simulink library "INP_DRVR"  (R2024b)
settings: Solver=VariableStepAuto  StartTime=0.0  StopTime=10.0  RelTol=1e-3
undefined symbols (not defined in the file or in its folder): p_RatSt_na
libraries: INP_DRVR_ManOver x1, INP_DRVR_Prep x1
settings Model: Creator=blatak  LastModifiedBy=jmbsp
settings ModelReferenceCC: EnableRefExpFcnMdlSchedulingChecks=on
settings RTWCC: GPUComputeCapability=3.5

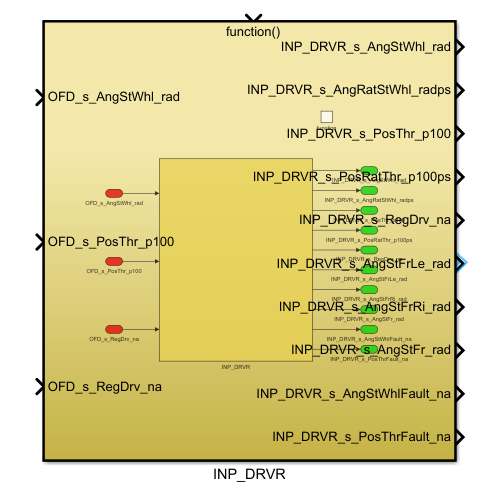
[thumbnail: Simulink's stored preview of the top-level diagram]
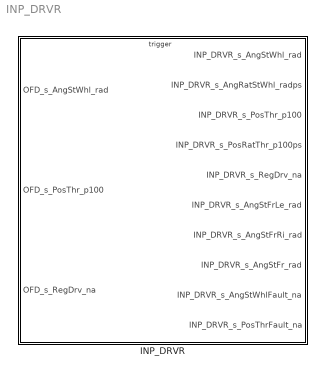
== system INP_DRVR ==
  INP_DRVR : Subsystem  Description=Driver actuation processing  TreatAsAtomicUnit=on

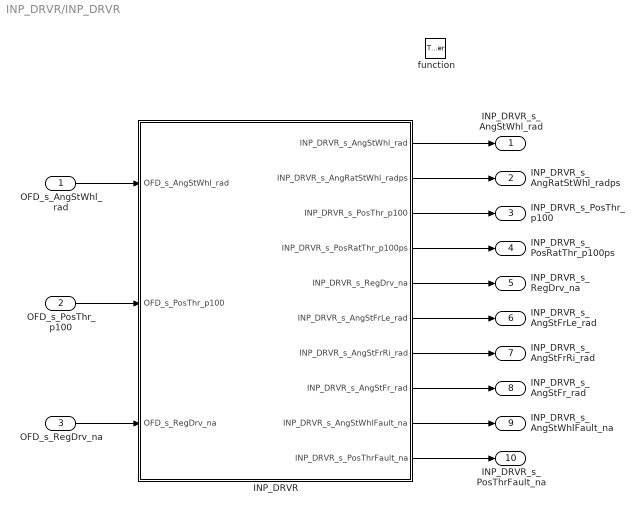
== system INP_DRVR/INP_DRVR ==
  OFD_s_AngStWhl_rad : Inport  Description=Steering wheel angle - raw measured value
  OFD_s_PosThr_p100 : Inport  Description=Throttle pedal position - raw measure value  Port=2
  OFD_s_RegDrv_na : Inport  Port=3
  function : TriggerPort  TriggerType=function-call  VariantControl=(inherit)
  INP_DRVR : Subsystem  Description=Driver actuation processing
  INP_DRVR_s_AngStWhl_rad : Outport  Description=INP Steering wheel angle - value after basic processing, filtering, scale, offset etc.
  INP_DRVR_s_AngRatStWhl_radps : Outport  Port=2
  INP_DRVR_s_PosThr_p100 : Outport  Description=INP Throttle pedal position - value after basic processing, filtering, scale, offset etc.  Port=3
  INP_DRVR_s_PosRatThr_p100ps : Outport  Port=4
  INP_DRVR_s_RegDrv_na : Outport  Port=5
  INP_DRVR_s_AngStFrLe_rad : Outport  Description=Steering wheel angle FL - calculated only from steering ratio (Ackerman neglected now)  Port=6
  INP_DRVR_s_AngStFrRi_rad : Outport  Description=Steering wheel angle FR - calculated only from steering ratio (Ackerman neglected now)  Port=7
  INP_DRVR_s_AngStFr_rad : Outport  Description=|  Port=8
      | Steering wheel angle front - calculated as an average FL and FR,
      | used for single track model, later more sophisticated calculation method needed 
      | than only an average
  INP_DRVR_s_AngStWhlFault_na : Outport  Port=9
  INP_DRVR_s_PosThrFault_na : Outport  Port=10
  wires:
  OFD_s_AngStWhl_rad/1 -> INP_DRVR/1(OFD_s_AngStWhl_rad)
  OFD_s_PosThr_p100/1 -> INP_DRVR/2(OFD_s_PosThr_p100)
  INP_DRVR/1(INP_DRVR_s_AngStWhl_rad) -> INP_DRVR_s_AngStWhl_rad/1
  INP_DRVR/3(INP_DRVR_s_PosThr_p100) -> INP_DRVR_s_PosThr_p100/1
  INP_DRVR/6(INP_DRVR_s_AngStFrLe_rad) -> INP_DRVR_s_AngStFrLe_rad/1
  INP_DRVR/7(INP_DRVR_s_AngStFrRi_rad) -> INP_DRVR_s_AngStFrRi_rad/1
  INP_DRVR/8(INP_DRVR_s_AngStFr_rad) -> INP_DRVR_s_AngStFr_rad/1
  INP_DRVR/2(INP_DRVR_s_AngRatStWhl_radps) -> INP_DRVR_s_AngRatStWhl_radps/1
  INP_DRVR/4(INP_DRVR_s_PosRatThr_p100ps) -> INP_DRVR_s_PosRatThr_p100ps/1
  INP_DRVR/9(INP_DRVR_s_AngStWhlFault_na) -> INP_DRVR_s_AngStWhlFault_na/1
  INP_DRVR/10(INP_DRVR_s_PosThrFault_na) -> INP_DRVR_s_PosThrFault_na/1
  OFD_s_RegDrv_na/1 -> INP_DRVR/3(OFD_s_RegDrv_na)
  INP_DRVR/5(INP_DRVR_s_RegDrv_na) -> INP_DRVR_s_RegDrv_na/1

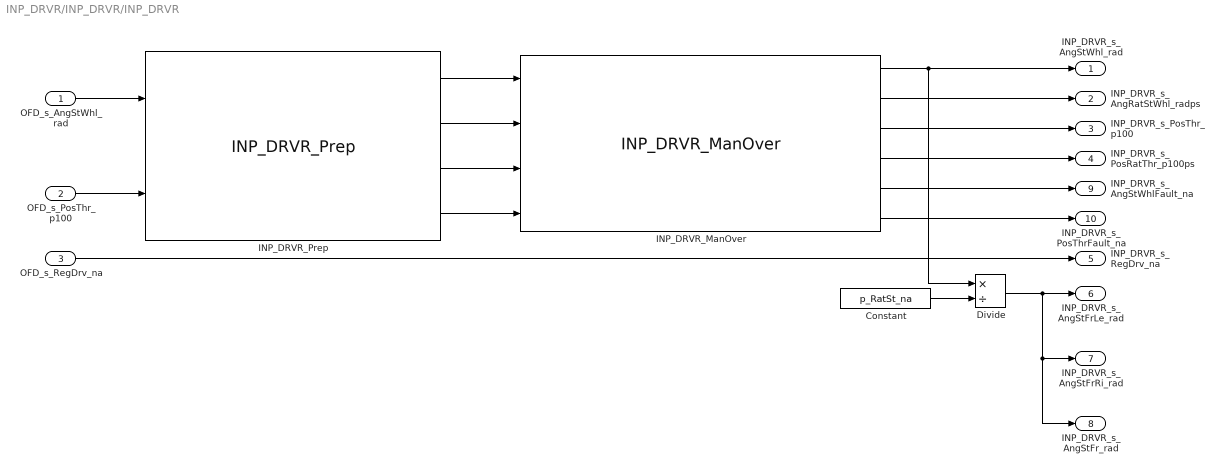
== system INP_DRVR/INP_DRVR/INP_DRVR ==
  OFD_s_AngStWhl_rad : Inport  Description=Steering wheel angle - raw measured value
  OFD_s_PosThr_p100 : Inport  Description=Throttle pedal position - raw measure value  Port=2
  OFD_s_RegDrv_na : Inport  Port=3
  Constant : Constant  Description=Steering ratio - the ratio between the steering wheel angle and the front steered wheels  Value=p_RatSt_na
  Divide : Product  Inputs=*/  RndMeth=Zero  SaturateOnIntegerOverflow=on
  INP_DRVR_ManOver : INP_DRVR_ManOver/INP_DRVR_ManOver  SystemSampleTime=-1  VariantActivationTime=update diagram  AllowFlexibleInterface=on  Latency=0  AutoFrameSizeCalculation=off
  INP_DRVR_Prep : INP_DRVR_Prep/INP_DRVR_Prep  SystemSampleTime=-1  VariantActivationTime=update diagram  AllowFlexibleInterface=on  Latency=0  AutoFrameSizeCalculation=off
  INP_DRVR_s_AngStWhl_rad : Outport  Description=INP Steering wheel angle - value after basic processing, filtering, scale, offset etc.
  INP_DRVR_s_AngRatStWhl_radps : Outport  Port=2
  INP_DRVR_s_PosThr_p100 : Outport  Description=INP Throttle pedal position - value after basic processing, filtering, scale, offset etc.  Port=3
  INP_DRVR_s_PosRatThr_p100ps : Outport  Port=4
  INP_DRVR_s_RegDrv_na : Outport  Port=5
  INP_DRVR_s_AngStFrLe_rad : Outport  Description=Steering wheel angle FL - calculated only from steering ratio (Ackerman neglected now)  Port=6
  INP_DRVR_s_AngStFrRi_rad : Outport  Description=Steering wheel angle FR - calculated only from steering ratio (Ackerman neglected now)  Port=7
  INP_DRVR_s_AngStFr_rad : Outport  Description=|  Port=8
      | Steering wheel angle front - calculated as an average FL and FR,
      | used for single track model, later more sophisticated calculation method needed 
      | than only an average
  INP_DRVR_s_AngStWhlFault_na : Outport  Port=9
  INP_DRVR_s_PosThrFault_na : Outport  Port=10
  wires:
  Constant/1 -> Divide/2
  Divide/1 -> INP_DRVR_s_AngStFr_rad/1, INP_DRVR_s_AngStFrRi_rad/1, INP_DRVR_s_AngStFrLe_rad/1
  OFD_s_PosThr_p100/1 -> INP_DRVR_Prep/2
  OFD_s_AngStWhl_rad/1 -> INP_DRVR_Prep/1
  INP_DRVR_Prep/1 -> INP_DRVR_ManOver/1
  INP_DRVR_Prep/2 -> INP_DRVR_ManOver/2
  INP_DRVR_Prep/3 -> INP_DRVR_ManOver/3
  INP_DRVR_Prep/4 -> INP_DRVR_ManOver/4
  INP_DRVR_ManOver/1 -> Divide/1, INP_DRVR_s_AngStWhl_rad/1
  INP_DRVR_ManOver/3 -> INP_DRVR_s_PosThr_p100/1
  INP_DRVR_ManOver/2 -> INP_DRVR_s_AngRatStWhl_radps/1
  INP_DRVR_ManOver/4 -> INP_DRVR_s_PosRatThr_p100ps/1
  INP_DRVR_ManOver/5 -> INP_DRVR_s_AngStWhlFault_na/1
  INP_DRVR_ManOver/6 -> INP_DRVR_s_PosThrFault_na/1
  OFD_s_RegDrv_na/1 -> INP_DRVR_s_RegDrv_na/1
